simulink model "ex2_2_2"  (Simulink 7.5)
settings: Solver=ode45  StartTime=0.0  StopTime=10.0  RelTol=1e-3
libraries: powerlib x8, powerlib_extras x3
settings Model: Creator=107108103  LastModifiedBy=Sambhav
settings OptimizationCC: InitFltsAndDblsToZero=on
settings DebuggingCC: StrictBusMsg=Warning

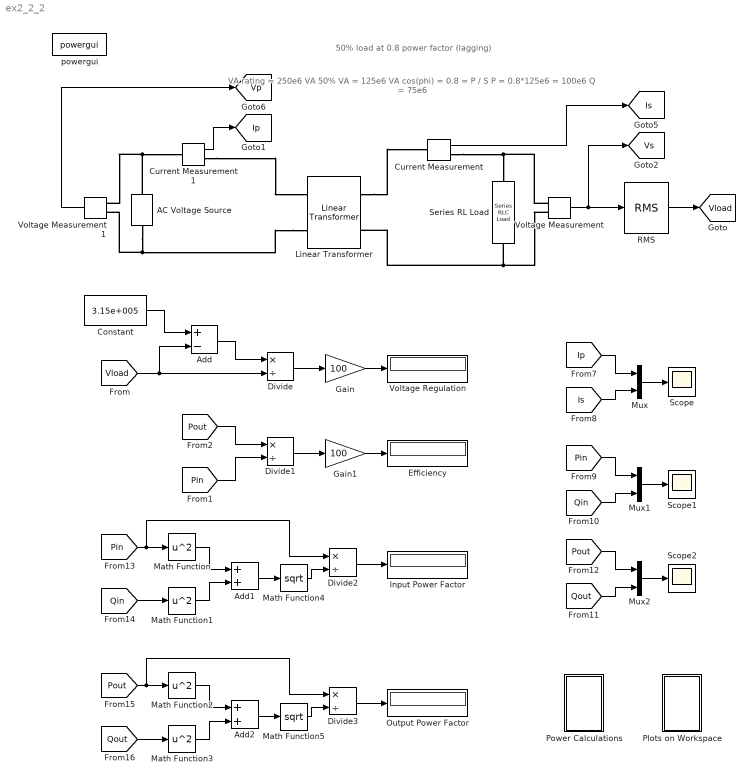
== system ex2_2_2 ==
  note: 50% load at 0.8 power factor (lagging)
  note: VA rating =  250e6 VA
      | 50% VA = 125e6 VA
      | cos(phi) = 0.8 = P / S
      | P = 0.8*125e6 = 100e6
      | Q = 75e6
  AC Voltage Source : powerlib/Electrical Sources/AC Voltage Source  DialogController=POWERSYS.PowerSysDialog  SystemSampleTime=-1  Amplitude=(7.35e+005)*sqrt(2)  Phase=0  Frequency=60  SampleTime=0  Measurements=None
  Add : Sum  Inputs=+-  OutDataType=sfix(16)  OutScaling=2^-10
  Add1 : Sum  OutDataType=sfix(16)  OutScaling=2^-10
  Add2 : Sum  OutDataType=sfix(16)  OutScaling=2^-10
  Constant : Constant  Value=3.15e+005  OutDataType=sfix(16)  OutScaling=2^0
  Current Measurement : powerlib/Measurements/Current Measurement  DialogController=POWERSYS.PowerSysDialog  SystemSampleTime=-1  PhasorSimulation=off  OutputType=Complex  PSBequivalent=0
  Current Measurement1 : powerlib/Measurements/Current Measurement  DialogController=POWERSYS.PowerSysDialog  SystemSampleTime=-1  PhasorSimulation=off  OutputType=Complex  PSBequivalent=0
  Divide{,1..3} (4 alike) : Product  Inputs=*/  OutDataType=sfix(16)  OutScaling=2^-10
  Efficiency : Display
  Gain : Gain  Gain=100  ParameterDataType=sfix(16)  ParameterScaling=2^0  OutDataType=sfix(16)  OutScaling=2^0
  Gain1 : Gain  Gain=100  ParameterDataType=sfix(16)  ParameterScaling=2^0  OutDataType=sfix(16)  OutScaling=2^0
  Input Power Factor : Display
  Linear Transformer : powerlib/Elements/Linear Transformer  DialogController=POWERSYS.PowerSysDialog  PhysicalDomain=powersysdomain  SubClassName=unknown  LeftPortType=p1  RightPortType=p1  LConnTagsString=a|b  RConnTagsString=A|B  UNITS=SI  NominalPower=[ 250e6 60 ]  winding1=[7.35e+005 4.3218 0.45856]  winding2=[3.15e+005 0.7938 0.084225]  ThreeWindings=off  winding3=[3.15e+005 0.7938 0.084225]  RmLm=[1.0805e+006 2866]  Measurements=None  DataType=on
  Math Function{,1..3} (4 alike) : Math  Operator=square  OutDataType=sfix(16)  OutScaling=2^0  SaturateOnIntegerOverflow=on
  Math Function4 : Math  Operator=sqrt  OutDataType=sfix(16)  OutScaling=2^0  SaturateOnIntegerOverflow=on
  Math Function5 : Math  Operator=sqrt  OutDataType=sfix(16)  OutScaling=2^0  SaturateOnIntegerOverflow=on
  Mux : Mux  Inputs=2
  Mux1 : Mux  Inputs=2
  Mux2 : Mux  Inputs=2
  Output Power Factor : Display
  Plots on Workspace : Subsystem
  Power Calculations : Subsystem
  RMS : powerlib_extras/Measurements/RMS  DialogController=POWERSYS.PowerSysDialog  SystemSampleTime=-1  f1=60
  Scope : Scope
  Scope1 : Scope
  Scope2 : Scope
      settings: SaveName=ScopeData2
  Series RL Load : powerlib/Elements/Series RLC Load  DialogController=POWERSYS.PowerSysDialog  PhysicalDomain=powersysdomain  SubClassName=unknown  LeftPortType=p1  RightPortType=p1  LConnTagsString=a  RConnTagsString=__new0  NominalVoltage=3.15e+005  NominalFrequency=60  ActivePower=100e6  InductivePower=75e6  CapacitivePower=0  Setx0=off  InitialVoltage=0  SetiL0=off  InitialCurrent=0  Measurements=None
  Voltage Measurement : powerlib/Measurements/Voltage Measurement  DialogController=POWERSYS.PowerSysDialog  SystemSampleTime=-1  PhasorSimulation=off  OutputType=Complex  PSBequivalent=0
  Voltage Measurement1 : powerlib/Measurements/Voltage Measurement  DialogController=POWERSYS.PowerSysDialog  SystemSampleTime=-1  PhasorSimulation=off  OutputType=Complex  PSBequivalent=0
  Voltage Regulation : Display
  powergui : powerlib/powergui  SystemSampleTime=-1  SimulationMode=Continuous  SampleTime=50e-6  frequency=60  SPID=off  DisableSnubberDevices=off  DisableRonSwitches=off  DisableVfSwitches=off  SwTol=0  Interpol=off  frequencyindice=60  echomessages=off  HookPort=off  DisplayEquations=off  FunctionMessages=off  EnableUseOfTLC=off  x0status=blocks  RestoreLinks=warning  ResistiveCurrentMeasurement=off  Frange=[0:2:500]  Ylog=off  Xlog=on  ShowGrid=off  save=off  variable=ZData  ZoomFFT=on  StartTime=0.0  cycles=1  DisplayStyle=1  fundamental=60  FreqAxis=off  MaxFrequency=1000  frequencyindicesteady=1  RmsSteady=1  display=off  Ts=0  methode=off
  tag scope: Ip=global, Is=global, Vload=global, Vp=global, Vs=global
  wires:
  Voltage Measurement/1 -> RMS/1, [Vs]
  RMS/1 -> [Vload]
  Gain1/1 -> Efficiency/1
  Divide1/1 -> Gain1/1
  [Pin] -> Divide1/2
  [Pout] -> Divide1/1
  Gain/1 -> Voltage Regulation/1
  Divide/1 -> Gain/1
  Add/1 -> Divide/1
  [Vload] -> Add/2, Divide/2
  Constant/1 -> Add/1
  Current Measurement/1 -> [Is]
  Current Measurement1/1 -> [Ip]
  Voltage Measurement1/1 -> [Vp]
  [Pin] -> Math Function/1, Divide2/1
  [Qin] -> Math Function1/1
  Math Function/1 -> Add1/1
  Math Function1/1 -> Add1/2
  Divide2/1 -> Input Power Factor/1
  [Pout] -> Divide3/1, Math Function2/1
  [Qout] -> Math Function3/1
  Math Function2/1 -> Add2/1
  Math Function3/1 -> Add2/2
  Divide3/1 -> Output Power Factor/1
  Add1/1 -> Math Function4/1
  Math Function4/1 -> Divide2/2
  Add2/1 -> Math Function5/1
  Math Function5/1 -> Divide3/2
  Mux1/1 -> Scope1/1
  [Qout] -> Mux2/2
  [Pout] -> Mux2/1
  [Qin] -> Mux1/2
  [Pin] -> Mux1/1
  Mux/1 -> Scope/1
  [Is] -> Mux/2
  [Ip] -> Mux/1
  Mux2/1 -> Scope2/1
  connections:
  Voltage Measurement/LConn1 -- Series RL Load/LConn1 -- Current Measurement/RConn1
  Voltage Measurement/LConn2 -- Linear Transformer/RConn2 -- Series RL Load/RConn1
  Linear Transformer/LConn2 -- AC Voltage Source/LConn1 -- Voltage Measurement1/LConn2
  Linear Transformer/RConn1 -- Current Measurement/LConn1
  AC Voltage Source/RConn1 -- Current Measurement1/LConn1 -- Voltage Measurement1/LConn1
  Current Measurement1/RConn1 -- Linear Transformer/LConn1

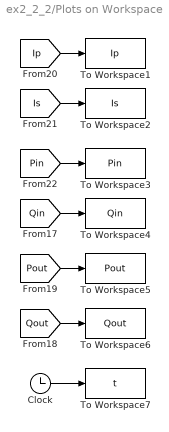
== system ex2_2_2/Plots on Workspace ==
  Clock : Clock
      settings: Decimation=10
  To Workspace1 : ToWorkspace  VariableName=Ip  SampleTime=-1  SaveFormat=Array
  To Workspace2 : ToWorkspace  VariableName=Is  SampleTime=-1  SaveFormat=Array
  To Workspace3 : ToWorkspace  VariableName=Pin  SampleTime=-1  SaveFormat=Array
  To Workspace4 : ToWorkspace  VariableName=Qin  SampleTime=-1  SaveFormat=Array
  To Workspace5 : ToWorkspace  VariableName=Pout  SampleTime=-1  SaveFormat=Array
  To Workspace6 : ToWorkspace  VariableName=Qout  SampleTime=-1  SaveFormat=Array
  To Workspace7 : ToWorkspace  VariableName=t  SampleTime=-1  SaveFormat=Array
  wires:
  Clock/1 -> To Workspace7/1
  [Ip] -> To Workspace1/1
  [Pin] -> To Workspace3/1
  [Qin] -> To Workspace4/1
  [Pout] -> To Workspace5/1
  [Qout] -> To Workspace6/1
  [Is] -> To Workspace2/1

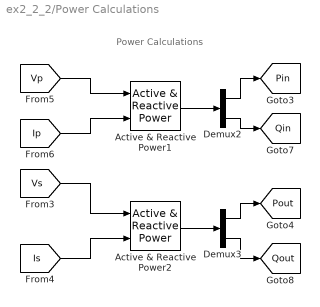
== system ex2_2_2/Power Calculations ==
  note: Power Calculations
  Active & Reactive Power1 : powerlib_extras/Measurements/Active & Reactive Power  DialogController=POWERSYS.PowerSysDialog  SystemSampleTime=-1  f1=60
  Active & Reactive Power2 : powerlib_extras/Measurements/Active & Reactive Power  DialogController=POWERSYS.PowerSysDialog  SystemSampleTime=-1  f1=60
  Demux2 : Demux  Outputs=2
  Demux3 : Demux  Outputs=2
  tag scope: Pin=global, Pout=global, Qin=global, Qout=global
  wires:
  [Vp] -> Active & Reactive Power1/1
  [Ip] -> Active & Reactive Power1/2
  [Is] -> Active & Reactive Power2/2
  [Vs] -> Active & Reactive Power2/1
  Demux3/1 -> [Pout]
  Active & Reactive Power2/1 -> Demux3/1
  Demux2/1 -> [Pin]
  Active & Reactive Power1/1 -> Demux2/1
  Demux2/2 -> [Qin]
  Demux3/2 -> [Qout]
